simulink model "MideaPMSM_V3_2019A"  (R2019b)
settings: Solver=ode4  StartTime=0.0  StopTime=0.2  FixedStep=1e-6  RelTol=1e-3
InitFcn:
  | Ts = 1e-6;
  | Pn = 3;
undefined symbols (not defined in the file or in its folder): DiscIntNeverNeededParam
libraries: powerlib x24, powerlib_extras x4, simulink x4, powerlib_meascontrol x3, dsparch4 x2
settings Model: Creator=B210b  LastModifiedBy=B210b
settings SFSimCC: CustomCodeUndefinedFunction=UseInterfaceOnly

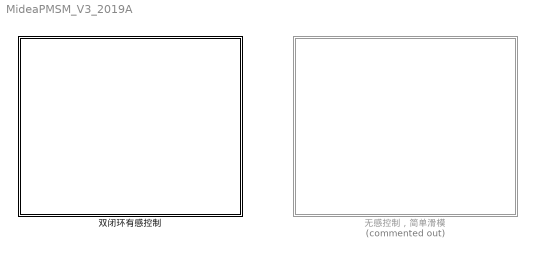
== system MideaPMSM_V3_2019A ==
  双闭环有感控制 : Subsystem
  无感控制，简单滑模 : Subsystem  Commented=on

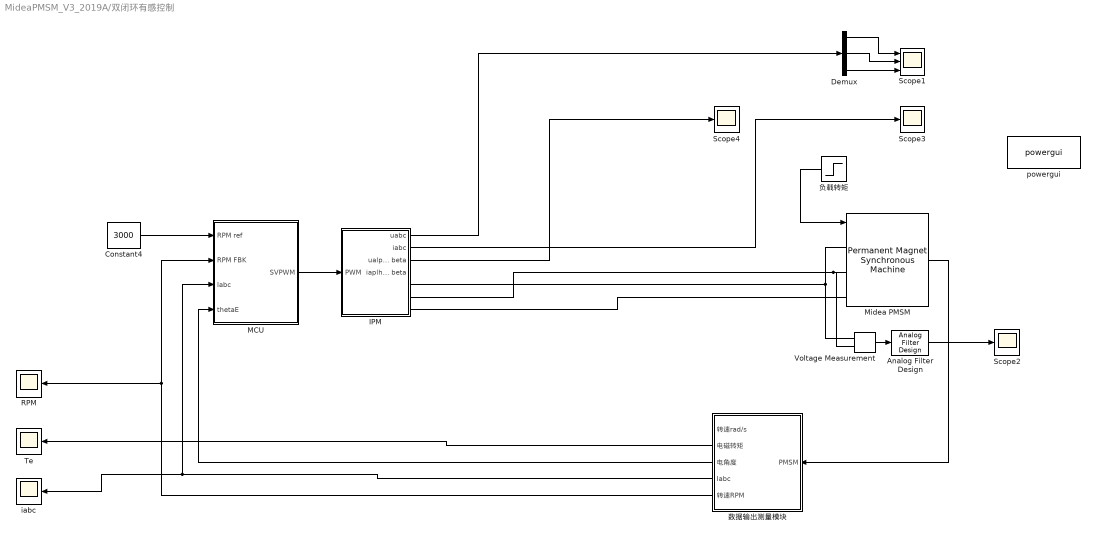
== system MideaPMSM_V3_2019A/双闭环有感控制 ==
  Analog Filter Design : dsparch4/Analog Filter Design  method=Butterworth  filttype=Lowpass  N=2  Wlo=30  Whi=80  Rp=2  Rs=40
  Constant4 : Constant  Value=3000
  Demux : Demux  Outputs=3
  IPM : Subsystem
  MCU : Subsystem
  Midea PMSM : powerlib/Machines/Permanent Magnet Synchronous Machine  NbPhases=3  FluxDistribution=Sinusoidal  RotorType=Salient-pole  MechanicalLoad=Torque Tm  PresetModel=No  ShowDetailedParameters=on  MeasurementBus=off  Resistance=26  Inductance=8.5e-3  dqInductances=[0.066 0.072]  La=0.000835  MachineConstant=Flux linkage established by magnets (V.s)  Flux=0.0714394  VoltageCst=38.873  TorqueCst=0.32148  Flat=120  Mechanical=[3.4e-05 0.000303448 3]  PolePairs=3  InitialConditions=[0,0, 0,0]  InitialConditions5ph=[0 0 0 0 0 0]  RefAngle=Aligned with phase A axis (original Park)  IterativeDiscreteModel=Trapezoidal non iterative  TsBlock=-1  TsPowergui=0
  RPM : Scope
  Scope1 : Scope  NumInputPorts=3
  Scope2 : Scope
  Scope3 : Scope
  Scope4 : Scope
  Te : Scope
  Voltage Measurement : powerlib/Measurements/Voltage Measurement  PhasorSimulation=off  OutputType=Complex  PSBequivalent=0
      settings: SourceProductName=Simscape Electrical
  iabc : Scope
  powergui : powerlib/powergui  SimulationMode=Discrete  SampleTime=1e-6  frequency=60  Iterations=50  frequencyindice=0  Pbase=100e6  ErrMax=1e-4  UnitsV=kV  UnitsW=MW  buscounter=0  FunctionMessages=off  echomessages=off  EnableUseOfTLC=off  CurrentSourceSwitches=on  DisableSnubberDevices=off  DisableRonSwitches=off  DisableVfSwitches=off  DisplayEquations=off  AutomaticDiscreteSolvers=off  SolverType=Tustin/Backward Euler (TBE)  Interpol=off  ExternalGateDelay=off  methode=off  Ts=0  x0status=blocks  SPID=off  SwTol=0  HookPort=off  NonlinearTolerance=1e-4  nMaxIteration=100  ContinueOnMaxIteration=off  RestoreLinks=warning  ResistiveCurrentMeasurement=off  Frange=[0:2:500]  Ylog=off  Xlog=on  ShowGrid=off  save=off  variable=ZData  structure=0  ZoomFFT=on  StartTime=0.0  cycles=1  DisplayStyle=1  fundamental=60  FreqAxis=off  MaxFrequency=1000  frequencyindicesteady=1  RmsSteady=1  display=off
      settings: SourceProductName=Simscape Electrical
  数据输出测量模块 : Subsystem
  负载转矩 : Step  Time=0.1  After=0  SampleTime=0
  wires:
  数据输出测量模块/3(电角度) -> MCU/4(thetaE)
  数据输出测量模块/5(转速RPM) -> MCU/2(RPM FBK), RPM/1
  负载转矩/1 -> Midea PMSM/1
  Midea PMSM/1 -> 数据输出测量模块/1(PMSM)
  数据输出测量模块/2(电磁转矩) -> Te/1
  Constant4/1 -> MCU/1(RPM ref)
  数据输出测量模块/4(Iabc) -> iabc/1, MCU/3(Iabc)
  MCU/1(SVPWM) -> IPM/1(PWM)
  IPM/2(iabc) -> Scope3/1
  IPM/3(ualpha beta) -> Scope4/1
  Demux/1 -> Scope1/1
  Demux/2 -> Scope1/2
  Demux/3 -> Scope1/3
  IPM/1(uabc) -> Demux/1
  Voltage Measurement/1 -> Analog Filter Design/1
  Analog Filter Design/1 -> Scope2/1
  connections:
  IPM/RConn3 -- Midea PMSM/LConn3
  IPM/RConn1 -- Midea PMSM/LConn1 -- Voltage Measurement/LConn1
  IPM/RConn2 -- Voltage Measurement/LConn2 -- Midea PMSM/LConn2

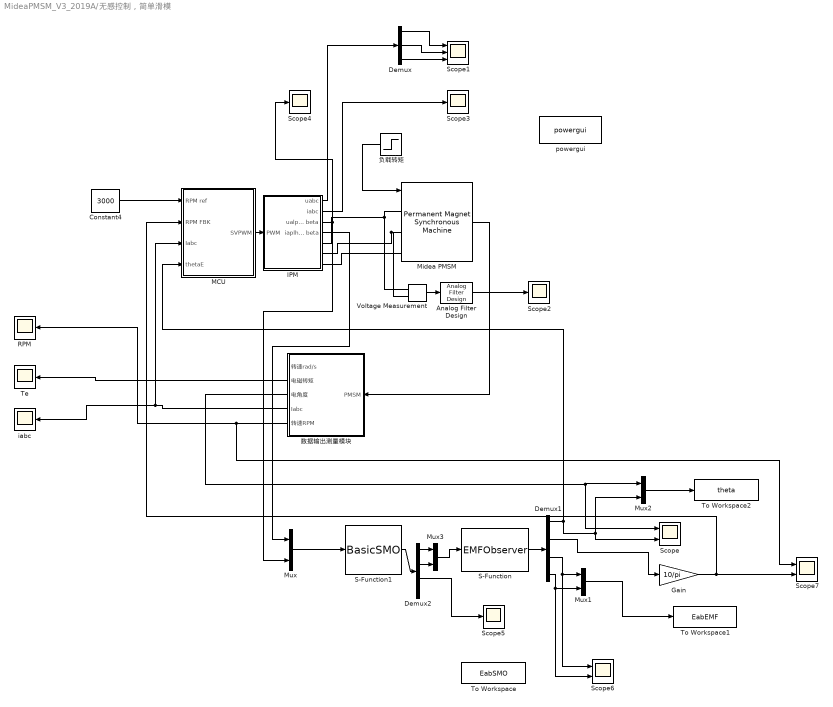
== system MideaPMSM_V3_2019A/无感控制，简单滑模 ==
  Analog Filter Design : dsparch4/Analog Filter Design  method=Butterworth  filttype=Lowpass  N=2  Wlo=30  Whi=80  Rp=2  Rs=40
  Constant4 : Constant  Value=3000
  Demux : Demux  Outputs=3
  Demux1 : Demux
  Demux2 : Demux
  Gain : Gain  Gain=10/pi
  IPM : Subsystem
  MCU : Subsystem
  Midea PMSM : powerlib/Machines/Permanent Magnet Synchronous Machine  NbPhases=3  FluxDistribution=Sinusoidal  RotorType=Round  MechanicalLoad=Torque Tm  PresetModel=No  ShowDetailedParameters=on  MeasurementBus=off  Resistance=26  Inductance=8.5e-3  dqInductances=[0.066 0.072]  La=0.0345  MachineConstant=Flux linkage established by magnets (V.s)  Flux=0.0779697  VoltageCst=42.4264  TorqueCst=0.35086  Flat=120  Mechanical=[3.4e-05 0 3]  PolePairs=3  InitialConditions=[0,0, 0,0]  InitialConditions5ph=[0 0 0 0 0 0]  RefAngle=Aligned with phase A axis (original Park)  IterativeDiscreteModel=Trapezoidal non iterative  TsBlock=-1  TsPowergui=0
  Mux{,1..3} (4 alike) : Mux  Inputs=2
  RPM : Scope
  S-Function : S-Function  FunctionName=EMFObserver  SFunctionDeploymentMode=off  EnableBusSupport=off
  S-Function1 : S-Function  FunctionName=BasicSMO  SFunctionDeploymentMode=off  EnableBusSupport=off
  Scope : Scope  NumInputPorts=2
  Scope1 : Scope  NumInputPorts=3
  Scope{2..5} (4 alike) : Scope
  Scope6 : Scope  NumInputPorts=2
  Scope7 : Scope  NumInputPorts=2
  Te : Scope
  To Workspace : ToWorkspace  VariableName=EabSMO  SaveFormat=Timeseries  SampleTime=-1
  To Workspace1 : ToWorkspace  VariableName=EabEMF  SaveFormat=Timeseries  SampleTime=-1
  To Workspace2 : ToWorkspace  VariableName=theta  SaveFormat=Timeseries  SampleTime=-1
  Voltage Measurement : powerlib/Measurements/Voltage Measurement  PhasorSimulation=off  OutputType=Complex  PSBequivalent=0
      settings: SourceProductName=Simscape Electrical
  iabc : Scope
  powergui : powerlib/powergui  SimulationMode=Discrete  SampleTime=1e-6  frequency=60  Iterations=50  frequencyindice=0  Pbase=100e6  ErrMax=1e-4  UnitsV=kV  UnitsW=MW  buscounter=0  FunctionMessages=off  echomessages=off  EnableUseOfTLC=off  CurrentSourceSwitches=on  DisableSnubberDevices=off  DisableRonSwitches=off  DisableVfSwitches=off  DisplayEquations=off  AutomaticDiscreteSolvers=off  SolverType=Tustin/Backward Euler (TBE)  Interpol=off  ExternalGateDelay=off  methode=off  Ts=0  x0status=blocks  SPID=off  SwTol=0  HookPort=off  NonlinearTolerance=1e-4  nMaxIteration=100  ContinueOnMaxIteration=off  RestoreLinks=warning  ResistiveCurrentMeasurement=off  Frange=[0:2:500]  Ylog=off  Xlog=on  ShowGrid=off  save=off  variable=ZData  structure=0  ZoomFFT=on  StartTime=0.0  cycles=1  DisplayStyle=1  fundamental=60  FreqAxis=off  MaxFrequency=1000  frequencyindicesteady=1  RmsSteady=1  display=off
      settings: SourceProductName=Simscape Electrical
  数据输出测量模块 : Subsystem
  负载转矩 : Step  Time=0.1  After=0.19  SampleTime=0
  wires:
  数据输出测量模块/3(电角度) -> Mux2/1, Scope/1
  负载转矩/1 -> Midea PMSM/1
  Midea PMSM/1 -> 数据输出测量模块/1(PMSM)
  数据输出测量模块/2(电磁转矩) -> Te/1
  Constant4/1 -> MCU/1(RPM ref)
  数据输出测量模块/4(Iabc) -> MCU/3(Iabc), iabc/1
  MCU/1(SVPWM) -> IPM/1(PWM)
  IPM/2(iabc) -> Scope3/1
  IPM/3(ualpha beta) -> Mux/2, Scope4/1
  Demux/1 -> Scope1/1
  Demux/2 -> Scope1/2
  Demux/3 -> Scope1/3
  IPM/1(uabc) -> Demux/1
  Voltage Measurement/1 -> Analog Filter Design/1
  Analog Filter Design/1 -> Scope2/1
  Mux/1 -> S-Function1/1
  IPM/4(iaplha beta) -> Mux/1
  S-Function/1 -> Demux1/1
  Demux1/4 -> Scope6/2, Mux1/2
  Demux1/3 -> Scope6/1, Mux1/1
  Demux1/2 -> Gain/1
  Gain/1 -> MCU/2(RPM FBK), Scope7/2
  Mux1/1 -> To Workspace1/1
  Mux2/1 -> To Workspace2/1
  Demux1/1 -> Scope/2, Mux2/2, MCU/4(thetaE)
  数据输出测量模块/5(转速RPM) -> Scope7/1, RPM/1
  S-Function1/1 -> Demux2/1
  Demux2/1 -> Mux3/1
  Demux2/2 -> Mux3/2
  Mux3/1 -> S-Function/1
  Demux2/3 -> Scope5/1
  connections:
  IPM/RConn3 -- Midea PMSM/LConn3
  IPM/RConn1 -- Midea PMSM/LConn1 -- Voltage Measurement/LConn1
  IPM/RConn2 -- Voltage Measurement/LConn2 -- Midea PMSM/LConn2

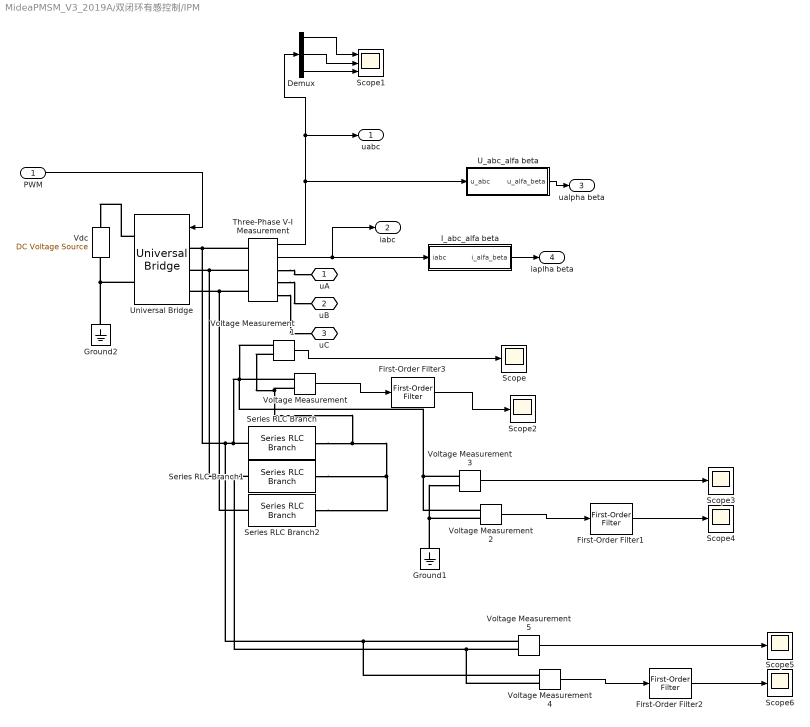
== system MideaPMSM_V3_2019A/双闭环有感控制/IPM ==
  PWM : Inport
  Demux : Demux  Outputs=3
  First-Order Filter1 : powerlib_meascontrol/Filters/First-Order Filter  FilterType=Lowpass  Tc=10e-3  Ts=0  Initialize=on  Vac_Init=[0, 0, 60]  Vdc_Init=0  PlotResponse=off  FreqRange="[0,  200,  1]"
      settings: SourceProductName=Simscape Electrical
  First-Order Filter2 : powerlib_meascontrol/Filters/First-Order Filter  FilterType=Lowpass  Tc=10e-3  Ts=0  Initialize=on  Vac_Init=[0, 0, 60]  Vdc_Init=0  PlotResponse=off  FreqRange="[0,  200,  1]"
      settings: SourceProductName=Simscape Electrical
  First-Order Filter3 : powerlib_meascontrol/Filters/First-Order Filter  FilterType=Lowpass  Tc=10e-3  Ts=0  Initialize=on  Vac_Init=[0, 0, 60]  Vdc_Init=0  PlotResponse=off  FreqRange="[0,  200,  1]"
      settings: SourceProductName=Simscape Electrical
  Ground1 : powerlib/Elements/Ground  LConnTagsString=a
      settings: SourceProductName=Simscape Electrical
  Ground2 : powerlib/Elements/Ground  LConnTagsString=a
      settings: SourceProductName=Simscape Electrical
  I_abc_alfa beta : Subsystem
  Scope{,2..6} (6 alike) : Scope
  Scope1 : Scope  NumInputPorts=3
  Series RLC Branch : powerlib/Elements/Series RLC Branch  LConnTagsString=__new0  RConnTagsString=__new0  BranchType=R  Resistance=5  Inductance=0  SetiL0=off  InitialCurrent=0  Capacitance=0  Setx0=off  InitialVoltage=0  Measurements=None
      settings: SourceProductName=Simscape Electrical
  Series RLC Branch1 : powerlib/Elements/Series RLC Branch  LConnTagsString=__new0  RConnTagsString=__new0  BranchType=R  Resistance=5  Inductance=0  SetiL0=off  InitialCurrent=0  Capacitance=0  Setx0=off  InitialVoltage=0  Measurements=None
      settings: SourceProductName=Simscape Electrical
  Series RLC Branch2 : powerlib/Elements/Series RLC Branch  LConnTagsString=__new0  RConnTagsString=__new0  BranchType=R  Resistance=5  Inductance=0  SetiL0=off  InitialCurrent=0  Capacitance=0  Setx0=off  InitialVoltage=0  Measurements=None
      settings: SourceProductName=Simscape Electrical
  Three-Phase V-I Measurement : powerlib/Measurements/Three-Phase V-I Measurement  VoltageMeasurement=phase-to-ground  SetLabelV=off  LabelV=Vabc  Vpu=off  VpuLL=off  CurrentMeasurement=yes  SetLabelI=off  LabelI=Iabc  Ipu=off  Pbase=100e6  Vbase=500e3  OutputType=Complex  PhasorSimulation=off  PSBequivalent=0
      settings: SourceProductName=Simscape Electrical
  U_abc_alfa beta : Subsystem
  Universal Bridge : powerlib/Power Electronics/Universal Bridge  Arms=3  SnubberResistance=1e5  SnubberCapacitance=inf  Device=IGBT / Diodes  Ron=1e-3  Lon=0  ForwardVoltages="[  0  0  ]"  ForwardVoltage=0  GTOparameters=[ 10e-6 , 20e-6 ]  IGBTparameters=[ 1e-6 , 2e-6 ]  Measurements=None  Measurements_2=None  converterType=Rectifier
      settings: SourceProductName=Simscape Electrical
  Vdc : powerlib/Electrical Sources/DC Voltage Source  Amplitude=311  Measurements=None
      settings: SourceProductName=Simscape Electrical
  Voltage Measurement{,1..5} (6 alike) : powerlib/Measurements/Voltage Measurement  PhasorSimulation=off  OutputType=Complex  PSBequivalent=0
      settings: SourceProductName=Simscape Electrical
  uA : PMIOPort  Side=Right
  uB : PMIOPort  Port=2  Side=Right
  uC : PMIOPort  Port=3  Side=Right
  uabc : Outport
  iabc : Outport  Port=2
  ualpha beta : Outport  Port=3
  iaplha beta : Outport  Port=4
  wires:
  PWM/1 -> Universal Bridge/1
  Three-Phase V-I Measurement/2 -> iabc/1, I_abc_alfa beta/1(iabc)
  I_abc_alfa beta/1(i_alfa_beta) -> iaplha beta/1
  U_abc_alfa beta/1(u_alfa_beta) -> ualpha beta/1
  Three-Phase V-I Measurement/1 -> U_abc_alfa beta/1(u_abc), Demux/1, uabc/1
  Voltage Measurement/1 -> First-Order Filter3/1
  Demux/2 -> Scope1/2
  Demux/1 -> Scope1/1
  Demux/3 -> Scope1/3
  Voltage Measurement1/1 -> Scope/1
  First-Order Filter1/1 -> Scope4/1
  Voltage Measurement3/1 -> Scope3/1
  Voltage Measurement2/1 -> First-Order Filter1/1
  First-Order Filter3/1 -> Scope2/1
  Voltage Measurement4/1 -> First-Order Filter2/1
  Voltage Measurement5/1 -> Scope5/1
  First-Order Filter2/1 -> Scope6/1
  connections:
  Universal Bridge/RConn1 -- Vdc/RConn1
  Universal Bridge/RConn2 -- Ground2/LConn1 -- Vdc/LConn1
  Three-Phase V-I Measurement/LConn1 -- Voltage Measurement4/LConn1 -- Voltage Measurement5/LConn1 -- Voltage Measurement2/LConn1 -- Voltage Measurement3/LConn1 -- Voltage Measurement1/LConn1 -- Voltage Measurement/LConn1 -- Series RLC Branch/LConn1 -- Universal Bridge/LConn1
  Three-Phase V-I Measurement/LConn2 -- Voltage Measurement4/LConn2 -- Voltage Measurement5/LConn2 -- Series RLC Branch1/LConn1 -- Universal Bridge/LConn2
  Three-Phase V-I Measurement/LConn3 -- Series RLC Branch2/LConn1 -- Universal Bridge/LConn3
  Three-Phase V-I Measurement/RConn1 -- uA/RConn1
  Three-Phase V-I Measurement/RConn2 -- uB/RConn1
  Three-Phase V-I Measurement/RConn3 -- uC/RConn1
  Series RLC Branch2/RConn1 -- Voltage Measurement1/LConn2 -- Voltage Measurement/LConn2 -- Series RLC Branch/RConn1 -- Series RLC Branch1/RConn1
  Ground1/LConn1 -- Voltage Measurement2/LConn2 -- Voltage Measurement3/LConn2

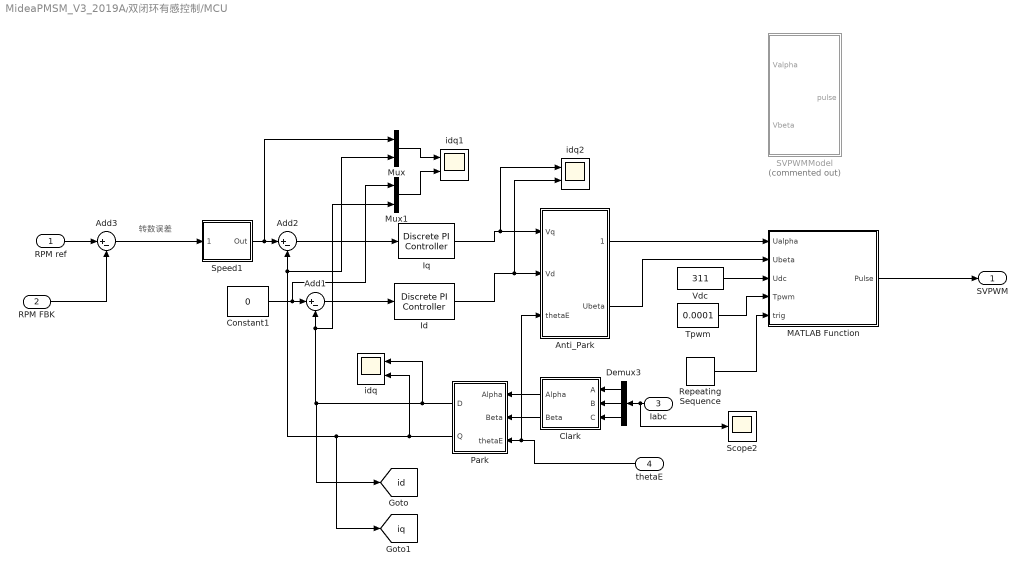
== system MideaPMSM_V3_2019A/双闭环有感控制/MCU ==
  note: 转数误差
  RPM ref : Inport
  RPM FBK : Inport  Port=2
  Iabc : Inport  Port=3
  thetaE : Inport  Port=4
  Add1 : Sum  Inputs=|+-
  Add2 : Sum  Inputs=|+-
  Add3 : Sum  Inputs=|+-
  Anti_Park : Subsystem
  Clark : Subsystem
  Constant1 : Constant  Value=0
  Demux3 : Demux  Outputs=3
  Id : powerlib_extras/Discrete  Control Blocks/Discrete PI Controller  Kp=500  Ki=100000  Par_Limits=[311*0.9*sqrt(3)/2 -311*0.9*sqrt(3)/2]  Init=0  Ts=Ts
      settings: SourceProductName=Simscape Electrical
  Iq : powerlib_extras/Discrete  Control Blocks/Discrete PI Controller  Kp=500  Ki=100000  Par_Limits=[311*0.9*sqrt(3)/2 -311*0.9*sqrt(3)/2]  Init=0  Ts=Ts
      settings: SourceProductName=Simscape Electrical
  MATLAB Function : MATLAB Function  TreatAsAtomicUnit=on
  Mux : Mux  Inputs=2
  Mux1 : Mux  Inputs=2
  Park : Subsystem
  Repeating Sequence : simulink/Sources/Repeating Sequence  rep_seq_t=[0 0.00005 0.0001]  rep_seq_y=[0 0.00005 0]
  SVPWMModel : Subsystem  Commented=on
  Scope2 : Scope
  Speed1 : Subsystem  AncestorBlock=|  DialogController=POWERSYS.PowerSysDialog  mask(Discrete PI Controller){Kpw=0.01, Kiw=2, Ba=0, Par_Limits=[2 -2], Init=0, Ts=-1}
      | powerlib_extras/Discrete 
      | Control Blocks/Discrete
      | PI Controller
      mask prompts: Kpw "Proportional gain (Kp):"; Kiw "Integral gain (Ki):"; Ba "feedback gain (Ba)"; Par_Limits "Output limits: [ Upper   Lower ]"; Init "Output initial value:"; Ts "Sample time:"
      mask help: This block implements a discrete PI controller.
      mask init:
      | UpperLimit=Par_Limits(1);
      | LowerLimit=Par_Limits(2);
      | power_initmask();
      mask Help: This block is part of a subset of blocks in the Extras library that does not have documentation associated with it, other than the block mask description.
      mask Display: disp('PI');
  Tpwm : Constant  Value=0.0001
  Vdc : Constant  Value=311
  idq : Scope  NumInputPorts=2
  idq1 : Scope  NumInputPorts=2
  idq2 : Scope  NumInputPorts=2
  SVPWM : Outport
  tag scope: id=global, iq=global
  wires:
  Clark/1(Alpha) -> Park/1(Alpha)
  Add1/1 -> Id/1
  Park/1(D) -> idq/1, [id], Mux1/2, Add1/2
  Iq/1 -> idq2/1, Anti_Park/1(Vq)
  Speed1/1(Out) -> Mux/1, Add2/1
  Park/2(Q) -> idq/2, [iq], Mux/2, Add2/2
  Id/1 -> idq2/2, Anti_Park/2(Vd)
  Demux3/3 -> Clark/3(C)
  Clark/2(Beta) -> Park/2(Beta)
  thetaE/1 -> Anti_Park/3(thetaE), Park/3(thetaE)
  Add2/1 -> Iq/1
  Demux3/1 -> Clark/1(A)
  Constant1/1 -> Mux1/1, Add1/1
  Demux3/2 -> Clark/2(B)
  Add3/1 -> Speed1/1(Error)
  Iabc/1 -> Scope2/1, Demux3/1
  RPM ref/1 -> Add3/1
  RPM FBK/1 -> Add3/2
  Mux/1 -> idq1/1
  Mux1/1 -> idq1/2
  Vdc/1 -> MATLAB Function/3(Udc)
  Tpwm/1 -> MATLAB Function/4(Tpwm)
  Anti_Park/1(Ualpha) -> MATLAB Function/1(Ualpha)
  Anti_Park/2(Ubeta) -> MATLAB Function/2(Ubeta)
  MATLAB Function/1(Pulse) -> SVPWM/1
  Repeating Sequence/1 -> MATLAB Function/5(trig)

== system MideaPMSM_V3_2019A/双闭环有感控制/数据输出测量模块 ==
  PMSM : Inport
  Mux : Subsystem
  Pn : Gain  Gain=Pn
  Scope : Scope  NumInputPorts=2
  wm->Nr : Gain  Gain=30/pi
  转速rad/s : Outport
  电磁转矩 : Outport  Port=2
  电角度 : Outport  Port=3
  Iabc : Outport  Port=4
  转速RPM : Outport  Port=5
  wires:
  Mux/1(Te) -> 电磁转矩/1
  Mux/2(The) -> Pn/1
  PMSM/1 -> Mux/1(m)
  Mux/4(Wm) -> wm->Nr/1, 转速rad/s/1
  Pn/1 -> 电角度/1
  Mux/3(Iabc) -> Iabc/1
  wm->Nr/1 -> 转速RPM/1
  Mux/5(vd) -> Scope/1
  Mux/6(vq) -> Scope/2

== system MideaPMSM_V3_2019A/无感控制，简单滑模/IPM ==
  PWM : Inport
  Ground2 : powerlib/Elements/Ground  LConnTagsString=a
      settings: SourceProductName=Simscape Electrical
  I_abc_alfa beta : Subsystem
  Three-Phase V-I Measurement : powerlib/Measurements/Three-Phase V-I Measurement  VoltageMeasurement=phase-to-ground  SetLabelV=off  LabelV=Vabc  Vpu=off  VpuLL=off  CurrentMeasurement=yes  SetLabelI=off  LabelI=Iabc  Ipu=off  Pbase=100e6  Vbase=500e3  OutputType=Complex  PhasorSimulation=off  PSBequivalent=0
      settings: SourceProductName=Simscape Electrical
  U_abc_alfa beta : Subsystem
  Universal Bridge : powerlib/Power Electronics/Universal Bridge  Arms=3  SnubberResistance=1e5  SnubberCapacitance=inf  Device=IGBT / Diodes  Ron=1e-3  Lon=0  ForwardVoltages="[  0  0  ]"  ForwardVoltage=0  GTOparameters=[ 10e-6 , 20e-6 ]  IGBTparameters=[ 1e-6 , 2e-6 ]  Measurements=None  Measurements_2=None  converterType=Rectifier
      settings: SourceProductName=Simscape Electrical
  Vdc : powerlib/Electrical Sources/DC Voltage Source  Amplitude=311  Measurements=None
      settings: SourceProductName=Simscape Electrical
  uA : PMIOPort  Side=Right
  uB : PMIOPort  Port=2  Side=Right
  uC : PMIOPort  Port=3  Side=Right
  uabc : Outport
  iabc : Outport  Port=2
  ualpha beta : Outport  Port=3
  iaplha beta : Outport  Port=4
  wires:
  PWM/1 -> Universal Bridge/1
  Three-Phase V-I Measurement/2 -> iabc/1, I_abc_alfa beta/1(iabc)
  I_abc_alfa beta/1(i_alfa_beta) -> iaplha beta/1
  U_abc_alfa beta/1(u_alfa_beta) -> ualpha beta/1
  Three-Phase V-I Measurement/1 -> U_abc_alfa beta/1(u_abc), uabc/1
  connections:
  Universal Bridge/RConn1 -- Vdc/RConn1
  Universal Bridge/RConn2 -- Ground2/LConn1 -- Vdc/LConn1
  Three-Phase V-I Measurement/LConn1 -- Universal Bridge/LConn1
  Three-Phase V-I Measurement/LConn2 -- Universal Bridge/LConn2
  Three-Phase V-I Measurement/LConn3 -- Universal Bridge/LConn3
  Three-Phase V-I Measurement/RConn1 -- uA/RConn1
  Three-Phase V-I Measurement/RConn2 -- uB/RConn1
  Three-Phase V-I Measurement/RConn3 -- uC/RConn1

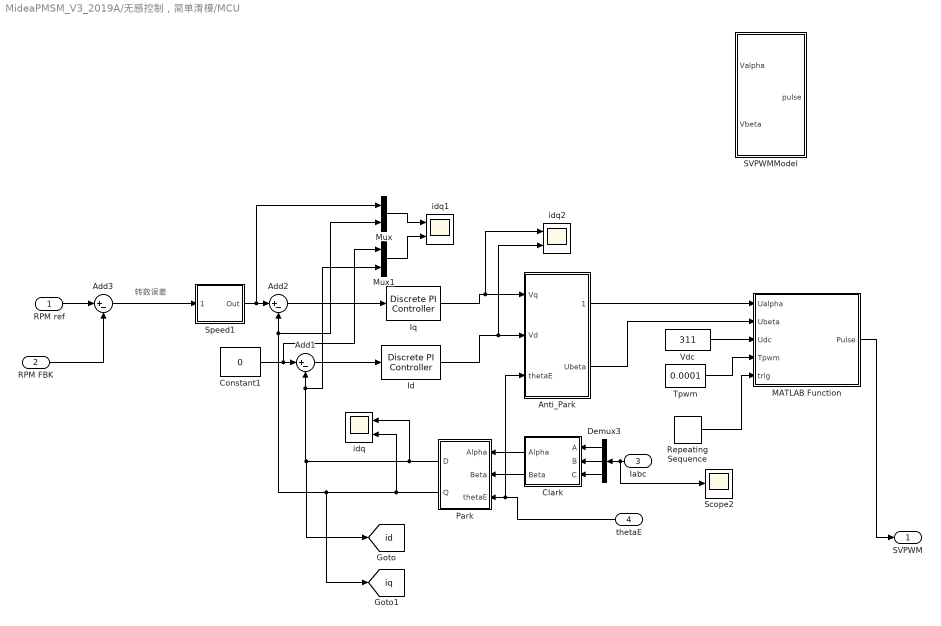
== system MideaPMSM_V3_2019A/无感控制，简单滑模/MCU ==
  note: 转数误差
  RPM ref : Inport
  RPM FBK : Inport  Port=2
  Iabc : Inport  Port=3
  thetaE : Inport  Port=4
  Add1 : Sum  Inputs=|+-
  Add2 : Sum  Inputs=|+-
  Add3 : Sum  Inputs=|+-
  Anti_Park : Subsystem
  Clark : Subsystem
  Constant1 : Constant  Value=0
  Demux3 : Demux  Outputs=3
  Id : powerlib_extras/Discrete  Control Blocks/Discrete PI Controller  Kp=500  Ki=100000  Par_Limits=[311*0.9*sqrt(3)/2 -311*0.9*sqrt(3)/2]  Init=0  Ts=Ts
      settings: SourceProductName=Simscape Electrical
  Iq : powerlib_extras/Discrete  Control Blocks/Discrete PI Controller  Kp=500  Ki=100000  Par_Limits=[311*0.9*sqrt(3)/2 -311*0.9*sqrt(3)/2]  Init=0  Ts=Ts
      settings: SourceProductName=Simscape Electrical
  MATLAB Function : MATLAB Function  TreatAsAtomicUnit=on
  Mux : Mux  Inputs=2
  Mux1 : Mux  Inputs=2
  Park : Subsystem
  Repeating Sequence : simulink/Sources/Repeating Sequence  rep_seq_t=[0 0.00005 0.0001]  rep_seq_y=[0 0.00005 0]
  SVPWMModel : Subsystem
  Scope2 : Scope
  Speed1 : Subsystem  AncestorBlock=|  DialogController=POWERSYS.PowerSysDialog  mask(Discrete PI Controller){Kpw=0.01, Kiw=2, Ba=0, Par_Limits=[2 -2], Init=0, Ts=-1}
      | powerlib_extras/Discrete 
      | Control Blocks/Discrete
      | PI Controller
      mask prompts: Kpw "Proportional gain (Kp):"; Kiw "Integral gain (Ki):"; Ba "feedback gain (Ba)"; Par_Limits "Output limits: [ Upper   Lower ]"; Init "Output initial value:"; Ts "Sample time:"
      mask help: This block implements a discrete PI controller.
      mask init:
      | UpperLimit=Par_Limits(1);
      | LowerLimit=Par_Limits(2);
      | power_initmask();
      mask Help: This block is part of a subset of blocks in the Extras library that does not have documentation associated with it, other than the block mask description.
      mask Display: disp('PI');
  Tpwm : Constant  Value=0.0001
  Vdc : Constant  Value=311
  idq : Scope  NumInputPorts=2
  idq1 : Scope  NumInputPorts=2
  idq2 : Scope  NumInputPorts=2
  SVPWM : Outport
  tag scope: id=global, iq=global
  wires:
  Clark/1(Alpha) -> Park/1(Alpha)
  Add1/1 -> Id/1
  Park/1(D) -> idq/1, [id], Mux1/2, Add1/2
  Iq/1 -> idq2/1, Anti_Park/1(Vq)
  Speed1/1(Out) -> Mux/1, Add2/1
  Park/2(Q) -> idq/2, [iq], Mux/2, Add2/2
  Id/1 -> idq2/2, Anti_Park/2(Vd)
  Demux3/3 -> Clark/3(C)
  Clark/2(Beta) -> Park/2(Beta)
  thetaE/1 -> Anti_Park/3(thetaE), Park/3(thetaE)
  Add2/1 -> Iq/1
  Demux3/1 -> Clark/1(A)
  Constant1/1 -> Mux1/1, Add1/1
  Demux3/2 -> Clark/2(B)
  Add3/1 -> Speed1/1(Error)
  Iabc/1 -> Scope2/1, Demux3/1
  RPM ref/1 -> Add3/1
  RPM FBK/1 -> Add3/2
  Mux/1 -> idq1/1
  Mux1/1 -> idq1/2
  Repeating Sequence/1 -> MATLAB Function/5(trig)
  Vdc/1 -> MATLAB Function/3(Udc)
  Tpwm/1 -> MATLAB Function/4(Tpwm)
  Anti_Park/1(Ualpha) -> MATLAB Function/1(Ualpha)
  Anti_Park/2(Ubeta) -> MATLAB Function/2(Ubeta)
  MATLAB Function/1(Pulse) -> SVPWM/1

== system MideaPMSM_V3_2019A/无感控制，简单滑模/数据输出测量模块 ==
  PMSM : Inport
  Constant : Constant  Value=2*pi
  Math Function : Math  Operator=rem  SignedPower=off  SaturateOnIntegerOverflow=on
  Mux : Subsystem
  Pn : Gain  Gain=Pn
  Scope : Scope  NumInputPorts=2
  wm->Nr : Gain  Gain=30/pi
  转速rad/s : Outport
  电磁转矩 : Outport  Port=2
  电角度 : Outport  Port=3
  Iabc : Outport  Port=4
  转速RPM : Outport  Port=5
  wires:
  Mux/1(Te) -> 电磁转矩/1
  Mux/2(The) -> Pn/1
  PMSM/1 -> Mux/1(m)
  Mux/4(Wm) -> wm->Nr/1, 转速rad/s/1
  Mux/3(Iabc) -> Iabc/1
  wm->Nr/1 -> 转速RPM/1
  Mux/5(vd) -> Scope/1
  Mux/6(vq) -> Scope/2
  Math Function/1 -> 电角度/1
  Pn/1 -> Math Function/1
  Constant/1 -> Math Function/2

== system MideaPMSM_V3_2019A/双闭环有感控制/IPM/I_abc_alfa beta ==
  iabc : Inport
  Fcn : Fcn  Expr=(2*u(1)-u(2)-u(3))/3
  Fcn1 : Fcn  Expr=(u(2)-u(3))/(3^(1/2))
  Mux2 : Mux  Inputs=2
  i_alfa_beta : Outport
  wires:
  iabc/1 -> Fcn/1, Fcn1/1
  Mux2/1 -> i_alfa_beta/1
  Fcn/1 -> Mux2/1
  Fcn1/1 -> Mux2/2

== system MideaPMSM_V3_2019A/双闭环有感控制/IPM/U_abc_alfa beta ==
  u_abc : Inport
  Fcn : Fcn  Expr=(2*u(1)-u(2)-u(3))/3
  Fcn1 : Fcn  Expr=(u(2)-u(3))/(3^(1/2))
  Mux2 : Mux  Inputs=2
  u_alfa_beta : Outport
  wires:
  u_abc/1 -> Fcn/1, Fcn1/1
  Mux2/1 -> u_alfa_beta/1
  Fcn/1 -> Mux2/1
  Fcn1/1 -> Mux2/2

== system MideaPMSM_V3_2019A/双闭环有感控制/MCU/Anti_Park ==
  Vq : Inport
  Vd : Inport  Port=2
  thetaE : Inport  Port=3
  Fcn : Fcn  Expr=cos(u[1])*u[2]-sin(u[1])*u[3]
  Fcn1 : Fcn  Expr=sin(u[1])*u[2]+cos(u[1])*u[3]
  Mux1 : Mux  Inputs=3
  Ualpha : Outport
  Ubeta : Outport  Port=2
  wires:
  Fcn1/1 -> Ubeta/1
  Fcn/1 -> Ualpha/1
  Mux1/1 -> Fcn/1, Fcn1/1
  Vd/1 -> Mux1/2
  Vq/1 -> Mux1/3
  thetaE/1 -> Mux1/1

== system MideaPMSM_V3_2019A/双闭环有感控制/MCU/Clark ==
  A : Inport
  B : Inport  Port=2
  C : Inport  Port=3
  Mux : Mux  Inputs=3
  alpha : Fcn  Expr=(u(1)-0.5*(u(2)+u(3)))*2/3
  beta : Fcn  Expr=sqrt(3)/2*(u(2)-u(3))*2/3
  Alpha : Outport
  Beta : Outport  Port=2
  wires:
  alpha/1 -> Alpha/1
  B/1 -> Mux/2
  C/1 -> Mux/3
  A/1 -> Mux/1
  Mux/1 -> beta/1, alpha/1
  beta/1 -> Beta/1

== system MideaPMSM_V3_2019A/双闭环有感控制/MCU/Park ==
  Alpha : Inport
  Beta : Inport  Port=2
  thetaE : Inport  Port=3
  Mux : Mux  Inputs=3
  d : Fcn  Expr=u(1)*cos(u(3))+u(2)*sin(u(3))
  q : Fcn  Expr=-u(1)*sin(u(3))+u(2)*cos(u(3))
  D : Outport
  Q : Outport  Port=2
  wires:
  d/1 -> D/1
  Beta/1 -> Mux/2
  Alpha/1 -> Mux/1
  Mux/1 -> q/1, d/1
  q/1 -> Q/1
  thetaE/1 -> Mux/3

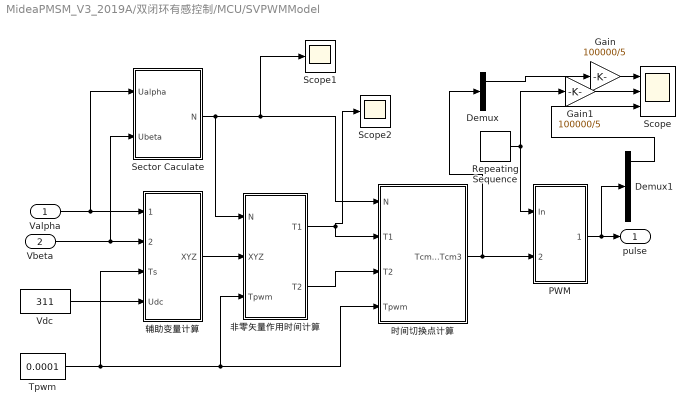
== system MideaPMSM_V3_2019A/双闭环有感控制/MCU/SVPWMModel ==
  Valpha : Inport
  Vbeta : Inport  Port=2
  Demux : Demux  Outputs=3
  Demux1 : Demux  Outputs=6
  Gain : Gain  Gain=100000/5
  Gain1 : Gain  Gain=100000/5
  PWM : Subsystem
  Repeating Sequence : simulink/Sources/Repeating Sequence  rep_seq_t=[0 0.00005 0.0001]  rep_seq_y=[0 0.00005 0]
  Scope : Scope  NumInputPorts=3
  Scope1 : Scope
  Scope2 : Scope
  Sector Caculate : Subsystem
  Tpwm : Constant  Value=0.0001
  Vdc : Constant  Value=311
  时间切换点计算 : Subsystem
  辅助变量计算 : Subsystem
  非零矢量作用时间计算 : Subsystem
  pulse : Outport
  wires:
  PWM/1(PWM) -> Demux1/1, pulse/1
  Repeating Sequence/1 -> Gain1/1, PWM/1(In)
  Vbeta/1 -> 辅助变量计算/2(Ubeta), Sector Caculate/2(Ubeta)
  非零矢量作用时间计算/1(T1) -> 时间切换点计算/2(T1), Scope2/1
  Valpha/1 -> 辅助变量计算/1(Ualpha), Sector Caculate/1(Ualpha)
  非零矢量作用时间计算/2(T2) -> 时间切换点计算/3(T2)
  Sector Caculate/1("N ") -> Scope1/1, 时间切换点计算/1(N), 非零矢量作用时间计算/1(N)
  辅助变量计算/1(XYZ) -> 非零矢量作用时间计算/2(XYZ)
  Tpwm/1 -> 辅助变量计算/3(Ts), 时间切换点计算/4(Tpwm), 非零矢量作用时间计算/3(Tpwm)
  Vdc/1 -> 辅助变量计算/4(Udc)
  时间切换点计算/1(Tcm1 Tcm2 Tcm3) -> PWM/2(Tcm123), Demux/1
  Demux/1 -> Gain/1
  Demux1/1 -> Scope/3
  Gain1/1 -> Scope/2
  Gain/1 -> Scope/1

== system MideaPMSM_V3_2019A/双闭环有感控制/MCU/Speed1 ==
  note: Discrete PID Controller
  note: Pierre Giroux, Gilbert Sybille
      | Power System Simulation Laboratory
      | IREQ, Hydro-Quebc
  Error : Inport  SampleTime=Ts
  Discrete-Time Integrator : DiscreteIntegrator  InitialCondition=Init  SampleTime=Ts  LimitOutput=on  UpperSaturationLimit=UpperLimit  LowerSaturationLimit=LowerLimit  ICPrevOutput=DiscIntNeverNeededParam  ICPrevScaledInput=DiscIntNeverNeededParam
  Kp1 : Gain  Gain=Ba  SampleTime=Ts  SaturateOnIntegerOverflow=on  OutDataTypeStr=Inherit: Same as input  ParamDataTypeStr=Inherit: Same as input
  Kp4 : Gain  Gain=Kpw  SampleTime=Ts  SaturateOnIntegerOverflow=on  OutDataTypeStr=Inherit: Same as input  ParamDataTypeStr=Inherit: Same as input
  Kp5 : Gain  Gain=Kiw  SampleTime=Ts  SaturateOnIntegerOverflow=on  OutDataTypeStr=Inherit: Same as input  ParamDataTypeStr=Inherit: Same as input
  Saturation2 : Saturate  UpperLimit=UpperLimit  LowerLimit=LowerLimit  SampleTime=Ts
  Sum6 : Sum  Inputs=++-  SampleTime=Ts  SaturateOnIntegerOverflow=on  InputSameDT=on  OutDataTypeStr=Inherit: Same as first input
  Zero-Order Hold : ZeroOrderHold  SampleTime=Ts
  Out : Outport  SampleTime=Ts  InitialOutput=0
  wires:
  Error/1 -> Kp1/1, Kp5/1, Kp4/1
  Zero-Order Hold/1 -> Sum6/1
  Saturation2/1 -> Out/1
  Discrete-Time Integrator/1 -> Sum6/2
  Kp4/1 -> Zero-Order Hold/1
  Kp5/1 -> Discrete-Time Integrator/1
  Sum6/1 -> Saturation2/1
  Kp1/1 -> Sum6/3

== system MideaPMSM_V3_2019A/双闭环有感控制/数据输出测量模块/Mux ==
  m : Inport
  Bus Selector : BusSelector  OutputSignals=Stator current is_a (A),Stator current is_b (A),Stator current is_c (A),Stator voltage Vs_q (V),Stator voltage Vs_d (V)
  Bus Selector1 : BusSelector  OutputSignals=Rotor speed wm (rad/s),Rotor angle thetam (rad),Electromagnetic torque Te (N*m)
  Mux : Mux  Inputs=3
  Te : Outport
  The : Outport  Port=2
  Iabc : Outport  Port=3
  Wm : Outport  Port=4
  vd : Outport  Port=5
  vq : Outport  Port=6
  wires:
  Bus Selector1/1 -> Wm/1  "<Rotor speed wm (rad/s)>"
  Bus Selector1/2 -> The/1  "<Rotor angle thetam (rad)>"
  Bus Selector1/3 -> Te/1  "<Electromagnetic torque Te (N*m)>"
  m/1 -> Bus Selector/1, Bus Selector1/1
  Bus Selector/2 -> Mux/2  "<Stator current is_b (A)>"
  Bus Selector/3 -> Mux/3  "<Stator current is_c (A)>"
  Bus Selector/1 -> Mux/1  "<Stator current is_a (A)>"
  Mux/1 -> Iabc/1
  Bus Selector/4 -> vq/1  "<Stator voltage Vs_q (V)>"
  Bus Selector/5 -> vd/1  "<Stator voltage Vs_d (V)>"

== system MideaPMSM_V3_2019A/无感控制，简单滑模/IPM/I_abc_alfa beta ==
  iabc : Inport
  Fcn : Fcn  Expr=(2*u(1)-u(2)-u(3))/3
  Fcn1 : Fcn  Expr=(u(2)-u(3))/(3^(1/2))
  Mux2 : Mux  Inputs=2
  i_alfa_beta : Outport
  wires:
  iabc/1 -> Fcn/1, Fcn1/1
  Mux2/1 -> i_alfa_beta/1
  Fcn/1 -> Mux2/1
  Fcn1/1 -> Mux2/2

== system MideaPMSM_V3_2019A/无感控制，简单滑模/IPM/U_abc_alfa beta ==
  u_abc : Inport
  Fcn : Fcn  Expr=(2*u(1)-u(2)-u(3))/3
  Fcn1 : Fcn  Expr=(u(2)-u(3))/(3^(1/2))
  Mux2 : Mux  Inputs=2
  u_alfa_beta : Outport
  wires:
  u_abc/1 -> Fcn/1, Fcn1/1
  Mux2/1 -> u_alfa_beta/1
  Fcn/1 -> Mux2/1
  Fcn1/1 -> Mux2/2

== system MideaPMSM_V3_2019A/无感控制，简单滑模/MCU/Anti_Park ==
  Vq : Inport
  Vd : Inport  Port=2
  thetaE : Inport  Port=3
  Fcn : Fcn  Expr=cos(u[1])*u[2]-sin(u[1])*u[3]
  Fcn1 : Fcn  Expr=sin(u[1])*u[2]+cos(u[1])*u[3]
  Mux1 : Mux  Inputs=3
  Ualpha : Outport
  Ubeta : Outport  Port=2
  wires:
  Fcn1/1 -> Ubeta/1
  Fcn/1 -> Ualpha/1
  Mux1/1 -> Fcn/1, Fcn1/1
  Vd/1 -> Mux1/2
  Vq/1 -> Mux1/3
  thetaE/1 -> Mux1/1

== system MideaPMSM_V3_2019A/无感控制，简单滑模/MCU/Clark ==
  A : Inport
  B : Inport  Port=2
  C : Inport  Port=3
  Mux : Mux  Inputs=3
  alpha : Fcn  Expr=(u(1)-0.5*(u(2)+u(3)))*2/3
  beta : Fcn  Expr=sqrt(3)/2*(u(2)-u(3))*2/3
  Alpha : Outport
  Beta : Outport  Port=2
  wires:
  alpha/1 -> Alpha/1
  B/1 -> Mux/2
  C/1 -> Mux/3
  A/1 -> Mux/1
  Mux/1 -> beta/1, alpha/1
  beta/1 -> Beta/1

== system MideaPMSM_V3_2019A/无感控制，简单滑模/MCU/Park ==
  Alpha : Inport
  Beta : Inport  Port=2
  thetaE : Inport  Port=3
  Mux : Mux  Inputs=3
  d : Fcn  Expr=u(1)*cos(u(3))+u(2)*sin(u(3))
  q : Fcn  Expr=-u(1)*sin(u(3))+u(2)*cos(u(3))
  D : Outport
  Q : Outport  Port=2
  wires:
  d/1 -> D/1
  Beta/1 -> Mux/2
  Alpha/1 -> Mux/1
  Mux/1 -> q/1, d/1
  q/1 -> Q/1
  thetaE/1 -> Mux/3

== system MideaPMSM_V3_2019A/无感控制，简单滑模/MCU/SVPWMModel ==
  Valpha : Inport
  Vbeta : Inport  Port=2
  PWM : Subsystem
  Repeating Sequence : simulink/Sources/Repeating Sequence  rep_seq_t=[0 0.00005 0.0001]  rep_seq_y=[0 0.00005 0]
  Sector Calculate : Subsystem
  T1T2 Calculate : Subsystem
  Tcm Calculate : Subsystem
  Tpwm : Constant  Value=0.0001
  Vdc : Constant  Value=311
  XYZ Calculate : Subsystem
  pulse : Outport
  wires:
  PWM/1(PWM) -> pulse/1
  Repeating Sequence/1 -> PWM/1(In)
  Vbeta/1 -> XYZ Calculate/2(Ubeta), Sector Calculate/2(Ubeta)
  T1T2 Calculate/1(T1) -> Tcm Calculate/2(T1)
  Valpha/1 -> XYZ Calculate/1(Ualpha), Sector Calculate/1(Ualpha)
  T1T2 Calculate/2(T2) -> Tcm Calculate/3(T2)
  Sector Calculate/1("N ") -> Tcm Calculate/1(N), T1T2 Calculate/1(N)
  XYZ Calculate/1(XYZ) -> T1T2 Calculate/2(XYZ)
  Tpwm/1 -> XYZ Calculate/3(Ts), Tcm Calculate/4(Tpwm), T1T2 Calculate/3(Tpwm)
  Vdc/1 -> XYZ Calculate/4(Udc)
  Tcm Calculate/1(Tcm1 Tcm2 Tcm3) -> PWM/2(Tcm123)

== system MideaPMSM_V3_2019A/无感控制，简单滑模/MCU/Speed1 ==
  note: Discrete PID Controller
  note: Pierre Giroux, Gilbert Sybille
      | Power System Simulation Laboratory
      | IREQ, Hydro-Quebc
  Error : Inport  SampleTime=Ts
  Discrete-Time Integrator : DiscreteIntegrator  InitialCondition=Init  SampleTime=Ts  LimitOutput=on  UpperSaturationLimit=UpperLimit  LowerSaturationLimit=LowerLimit  ICPrevOutput=DiscIntNeverNeededParam  ICPrevScaledInput=DiscIntNeverNeededParam
  Kp1 : Gain  Gain=Ba  SampleTime=Ts  SaturateOnIntegerOverflow=on  OutDataTypeStr=Inherit: Same as input  ParamDataTypeStr=Inherit: Same as input
  Kp4 : Gain  Gain=Kpw  SampleTime=Ts  SaturateOnIntegerOverflow=on  OutDataTypeStr=Inherit: Same as input  ParamDataTypeStr=Inherit: Same as input
  Kp5 : Gain  Gain=Kiw  SampleTime=Ts  SaturateOnIntegerOverflow=on  OutDataTypeStr=Inherit: Same as input  ParamDataTypeStr=Inherit: Same as input
  Saturation2 : Saturate  UpperLimit=UpperLimit  LowerLimit=LowerLimit  SampleTime=Ts
  Sum6 : Sum  Inputs=++-  SampleTime=Ts  SaturateOnIntegerOverflow=on  InputSameDT=on  OutDataTypeStr=Inherit: Same as first input
  Zero-Order Hold : ZeroOrderHold  SampleTime=Ts
  Out : Outport  SampleTime=Ts  InitialOutput=0
  wires:
  Error/1 -> Kp1/1, Kp5/1, Kp4/1
  Zero-Order Hold/1 -> Sum6/1
  Saturation2/1 -> Out/1
  Discrete-Time Integrator/1 -> Sum6/2
  Kp4/1 -> Zero-Order Hold/1
  Kp5/1 -> Discrete-Time Integrator/1
  Sum6/1 -> Saturation2/1
  Kp1/1 -> Sum6/3

== system MideaPMSM_V3_2019A/无感控制，简单滑模/数据输出测量模块/Mux ==
  m : Inport
  Bus Selector : BusSelector  OutputSignals=Stator current is_a (A),Stator current is_b (A),Stator current is_c (A),Stator voltage Vs_q (V),Stator voltage Vs_d (V)
  Bus Selector1 : BusSelector  OutputSignals=Rotor speed wm (rad/s),Rotor angle thetam (rad),Electromagnetic torque Te (N*m)
  Mux : Mux  Inputs=3
  Te : Outport
  The : Outport  Port=2
  Iabc : Outport  Port=3
  Wm : Outport  Port=4
  vd : Outport  Port=5
  vq : Outport  Port=6
  wires:
  Bus Selector1/1 -> Wm/1  "<Rotor speed wm (rad/s)>"
  Bus Selector1/2 -> The/1  "<Rotor angle thetam (rad)>"
  Bus Selector1/3 -> Te/1  "<Electromagnetic torque Te (N*m)>"
  m/1 -> Bus Selector/1, Bus Selector1/1
  Bus Selector/2 -> Mux/2  "<Stator current is_b (A)>"
  Bus Selector/3 -> Mux/3  "<Stator current is_c (A)>"
  Bus Selector/1 -> Mux/1  "<Stator current is_a (A)>"
  Mux/1 -> Iabc/1
  Bus Selector/4 -> vq/1  "<Stator voltage Vs_q (V)>"
  Bus Selector/5 -> vd/1  "<Stator voltage Vs_d (V)>"

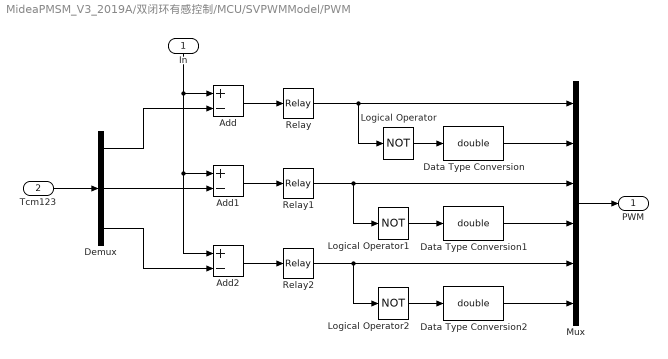
== system MideaPMSM_V3_2019A/双闭环有感控制/MCU/SVPWMModel/PWM ==
  In : Inport
  Tcm123 : Inport  Port=2
  Add : Sum  Inputs=+-
  Add1 : Sum  Inputs=+-
  Add2 : Sum  Inputs=+-
  Data Type Conversion : DataTypeConversion  OutDataTypeStr=double
  Data Type Conversion1 : DataTypeConversion  OutDataTypeStr=double
  Data Type Conversion2 : DataTypeConversion  OutDataTypeStr=double
  Demux : Demux  Outputs=3
  Logical Operator : Logic  Operator=NOT  AllPortsSameDT=off  OutDataTypeStr=boolean
  Logical Operator1 : Logic  Operator=NOT  AllPortsSameDT=off  OutDataTypeStr=boolean
  Logical Operator2 : Logic  Operator=NOT  AllPortsSameDT=off  OutDataTypeStr=boolean
  Mux : Mux  Inputs=6
  Relay : Relay  OffSwitchValue=-eps
  Relay1 : Relay  OffSwitchValue=-eps
  Relay2 : Relay  OffSwitchValue=-eps
  PWM : Outport
  wires:
  Demux/3 -> Add2/2
  Demux/2 -> Add1/2
  Demux/1 -> Add/2
  Relay2/1 -> Mux/5, Logical Operator2/1
  Relay1/1 -> Mux/3, Logical Operator1/1
  Relay/1 -> Logical Operator/1, Mux/1
  Mux/1 -> PWM/1
  Data Type Conversion/1 -> Mux/2
  Data Type Conversion1/1 -> Mux/4
  Data Type Conversion2/1 -> Mux/6
  Logical Operator2/1 -> Data Type Conversion2/1
  Logical Operator1/1 -> Data Type Conversion1/1
  Logical Operator/1 -> Data Type Conversion/1
  Add1/1 -> Relay1/1
  Add2/1 -> Relay2/1
  Add/1 -> Relay/1
  In/1 -> Add/1, Add2/1, Add1/1
  Tcm123/1 -> Demux/1

== system MideaPMSM_V3_2019A/双闭环有感控制/MCU/SVPWMModel/Sector Caculate ==
  Ualpha : Inport
  Ubeta : Inport  Port=2
  B0 : Fcn  Expr=u[2]
  B1 : Fcn  Expr=u[1]*sqrt(3/4)-0.5*u[2]
  B2 : Fcn  Expr=-u[1]*sqrt(3/4)-u[2]*0.5
  Constant : Constant
  Constant1 : Constant  Value=0
  Mux : Mux  Inputs=2
  Mux1 : Mux  Inputs=3
  N : Fcn  Expr=4*u[3]+2*u[2]+u[1]
  Switch : Switch
  Switch1 : Switch
  Switch2 : Switch
  "N " : Outport
  wires:
  Switch2/1 -> Mux1/3
  Switch/1 -> Mux1/1
  Ualpha/1 -> Mux/1
  Ubeta/1 -> Mux/2
  Mux/1 -> B2/1, B1/1, B0/1
  B0/1 -> Switch/2
  B1/1 -> Switch1/2
  B2/1 -> Switch2/2
  Constant/1 -> Switch/1, Switch2/1, Switch1/1
  Constant1/1 -> Switch/3, Switch1/3, Switch2/3
  Switch1/1 -> Mux1/2
  Mux1/1 -> N/1
  N/1 -> "N "/1

== system MideaPMSM_V3_2019A/双闭环有感控制/MCU/SVPWMModel/时间切换点计算 ==
  N : Inport
  T1 : Inport  Port=2
  T2 : Inport  Port=3
  Tpwm : Inport  Port=4
  Fcn : Fcn  Expr=(u[3]-u[1]-u[2])/4
  Fcn1 : Fcn  Expr=(u[3]+u[1]-u[2])/4
  Fcn2 : Fcn  Expr=(u[3]+u[2]+u[1])/4
  Multiport Switch : MultiPortSwitch  Inputs=6
  Multiport Switch1 : MultiPortSwitch  Inputs=6
  Multiport Switch2 : MultiPortSwitch  Inputs=6
  Mux : Mux  Inputs=3
  Mux1 : Mux  Inputs=3
  Tcm1 Tcm2 Tcm3 : Outport
  wires:
  Mux/1 -> Fcn2/1, Fcn/1, Fcn1/1
  Tpwm/1 -> Mux/3
  T2/1 -> Mux/2
  T1/1 -> Mux/1
  Multiport Switch2/1 -> Mux1/3
  Multiport Switch1/1 -> Mux1/2
  Multiport Switch/1 -> Mux1/1
  Mux1/1 -> Tcm1 Tcm2 Tcm3/1
  Fcn/1 -> Multiport Switch/3, Multiport Switch/4, Multiport Switch1/6, Multiport Switch2/5, Multiport Switch2/7, Multiport Switch1/2
  Fcn1/1 -> Multiport Switch1/5, Multiport Switch2/3, Multiport Switch2/6, Multiport Switch1/4, Multiport Switch/7, Multiport Switch/2
  Fcn2/1 -> Multiport Switch/5, Multiport Switch/6, Multiport Switch1/3, Multiport Switch1/7, Multiport Switch2/2, Multiport Switch2/4
  N/1 -> Multiport Switch2/1, Multiport Switch1/1, Multiport Switch/1

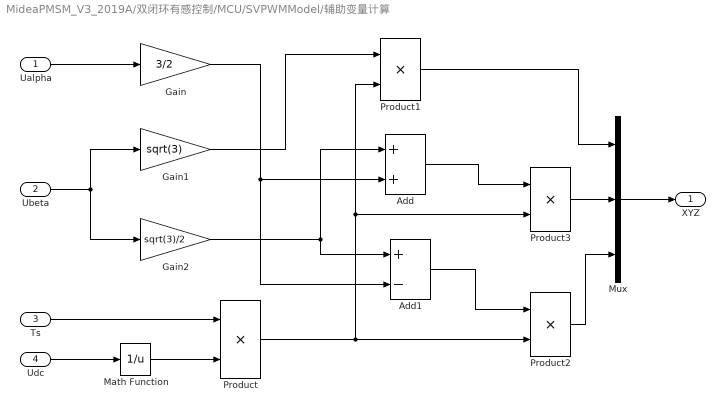
== system MideaPMSM_V3_2019A/双闭环有感控制/MCU/SVPWMModel/辅助变量计算 ==
  Ualpha : Inport
  Ubeta : Inport  Port=2
  Ts : Inport  Port=3
  Udc : Inport  Port=4
  Add : Sum
  Add1 : Sum  Inputs=+-
  Gain : Gain  Gain=3/2
  Gain1 : Gain  Gain=sqrt(3)
  Gain2 : Gain  Gain=sqrt(3)/2
  Math Function : Math  Operator=reciprocal  SaturateOnIntegerOverflow=on
  Mux : Mux  Inputs=3
  Product{,1..3} (4 alike) : Product  RndMeth=Zero
  XYZ : Outport
  wires:
  Mux/1 -> XYZ/1
  Product1/1 -> Mux/1
  Product3/1 -> Mux/2
  Product2/1 -> Mux/3
  Ualpha/1 -> Gain/1
  Ubeta/1 -> Gain2/1, Gain1/1
  Udc/1 -> Math Function/1
  Math Function/1 -> Product/2
  Ts/1 -> Product/1
  Gain1/1 -> Product1/1
  Product/1 -> Product2/2, Product1/2, Product3/2
  Gain/1 -> Add1/2, Add/2
  Gain2/1 -> Add/1, Add1/1
  Add1/1 -> Product2/1
  Add/1 -> Product3/1

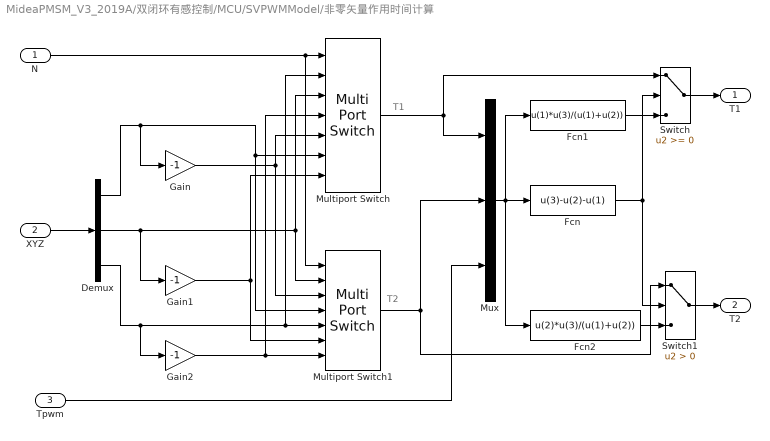
== system MideaPMSM_V3_2019A/双闭环有感控制/MCU/SVPWMModel/非零矢量作用时间计算 ==
  note: T1
  note: T2
  N : Inport
  XYZ : Inport  Port=2
  Tpwm : Inport  Port=3
  Demux : Demux  Outputs=3
  Fcn : Fcn  Expr=u(3)-u(2)-u(1)
  Fcn1 : Fcn  Expr=u(1)*u(3)/(u(1)+u(2))
  Fcn2 : Fcn  Expr=u(2)*u(3)/(u(1)+u(2))
  Gain : Gain  Gain=-1
  Gain1 : Gain  Gain=-1
  Gain2 : Gain  Gain=-1
  Multiport Switch : MultiPortSwitch  Inputs=6
  Multiport Switch1 : MultiPortSwitch  Inputs=6
  Mux : Mux  Inputs=3
  Switch : Switch
  Switch1 : Switch  Criteria=u2 > Threshold
  T1 : Outport
  T2 : Outport  Port=2
  wires:
  Tpwm/1 -> Mux/3
  XYZ/1 -> Demux/1
  Switch1/1 -> T2/1
  Switch/1 -> T1/1
  Fcn2/1 -> Switch1/3
  Fcn1/1 -> Switch/3
  Fcn/1 -> Switch/2, Switch1/2
  Mux/1 -> Fcn1/1, Fcn/1, Fcn2/1
  Multiport Switch/1 -> Switch/1, Mux/1
  Multiport Switch1/1 -> Switch1/1, Mux/2
  N/1 -> Multiport Switch/1, Multiport Switch1/1
  Demux/2 -> Multiport Switch/3, Multiport Switch1/2, Gain1/1
  Demux/3 -> Multiport Switch1/5, Multiport Switch/2, Gain2/1
  Demux/1 -> Multiport Switch/6, Multiport Switch1/4, Gain/1
  Gain/1 -> Multiport Switch1/3, Multiport Switch/5
  Gain2/1 -> Multiport Switch/4, Multiport Switch1/7
  Gain1/1 -> Multiport Switch1/6, Multiport Switch/7

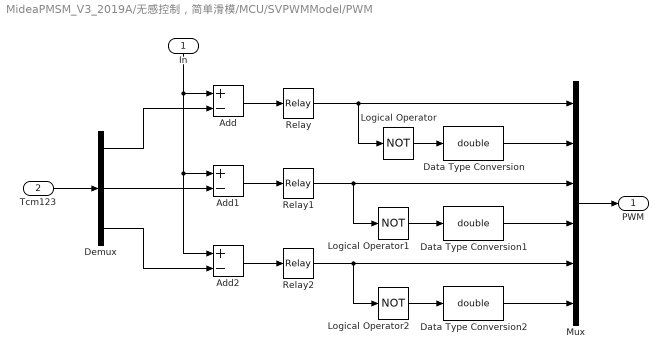
== system MideaPMSM_V3_2019A/无感控制，简单滑模/MCU/SVPWMModel/PWM ==
  In : Inport
  Tcm123 : Inport  Port=2
  Add : Sum  Inputs=+-
  Add1 : Sum  Inputs=+-
  Add2 : Sum  Inputs=+-
  Data Type Conversion : DataTypeConversion  OutDataTypeStr=double
  Data Type Conversion1 : DataTypeConversion  OutDataTypeStr=double
  Data Type Conversion2 : DataTypeConversion  OutDataTypeStr=double
  Demux : Demux  Outputs=3
  Logical Operator : Logic  Operator=NOT  AllPortsSameDT=off  OutDataTypeStr=boolean
  Logical Operator1 : Logic  Operator=NOT  AllPortsSameDT=off  OutDataTypeStr=boolean
  Logical Operator2 : Logic  Operator=NOT  AllPortsSameDT=off  OutDataTypeStr=boolean
  Mux : Mux  Inputs=6
  Relay : Relay  OffSwitchValue=-eps
  Relay1 : Relay  OffSwitchValue=-eps
  Relay2 : Relay  OffSwitchValue=-eps
  PWM : Outport
  wires:
  Demux/3 -> Add2/2
  Demux/2 -> Add1/2
  Demux/1 -> Add/2
  Relay2/1 -> Mux/5, Logical Operator2/1
  Relay1/1 -> Mux/3, Logical Operator1/1
  Relay/1 -> Logical Operator/1, Mux/1
  Mux/1 -> PWM/1
  Data Type Conversion/1 -> Mux/2
  Data Type Conversion1/1 -> Mux/4
  Data Type Conversion2/1 -> Mux/6
  Logical Operator2/1 -> Data Type Conversion2/1
  Logical Operator1/1 -> Data Type Conversion1/1
  Logical Operator/1 -> Data Type Conversion/1
  Add1/1 -> Relay1/1
  Add2/1 -> Relay2/1
  Add/1 -> Relay/1
  In/1 -> Add/1, Add2/1, Add1/1
  Tcm123/1 -> Demux/1

== system MideaPMSM_V3_2019A/无感控制，简单滑模/MCU/SVPWMModel/Sector Calculate ==
  Ualpha : Inport
  Ubeta : Inport  Port=2
  B0 : Fcn  Expr=u[2]
  B1 : Fcn  Expr=u[1]*sqrt(3/4)-0.5*u[2]
  B2 : Fcn  Expr=-u[1]*sqrt(3/4)-u[2]*0.5
  Constant : Constant
  Constant1 : Constant  Value=0
  Mux : Mux  Inputs=2
  Mux1 : Mux  Inputs=3
  N : Fcn  Expr=4*u[3]+2*u[2]+u[1]
  Switch : Switch
  Switch1 : Switch
  Switch2 : Switch
  "N " : Outport
  wires:
  Switch2/1 -> Mux1/3
  Switch/1 -> Mux1/1
  Ualpha/1 -> Mux/1
  Ubeta/1 -> Mux/2
  Mux/1 -> B2/1, B1/1, B0/1
  B0/1 -> Switch/2
  B1/1 -> Switch1/2
  B2/1 -> Switch2/2
  Constant/1 -> Switch/1, Switch2/1, Switch1/1
  Constant1/1 -> Switch/3, Switch1/3, Switch2/3
  Switch1/1 -> Mux1/2
  Mux1/1 -> N/1
  N/1 -> "N "/1

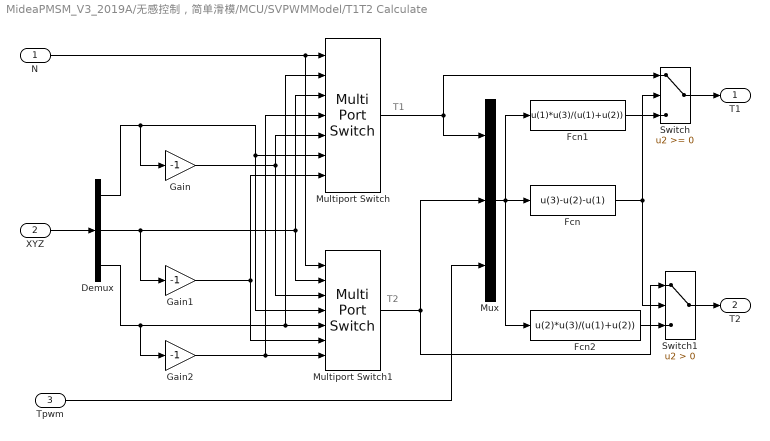
== system MideaPMSM_V3_2019A/无感控制，简单滑模/MCU/SVPWMModel/T1T2 Calculate ==
  note: T1
  note: T2
  N : Inport
  XYZ : Inport  Port=2
  Tpwm : Inport  Port=3
  Demux : Demux  Outputs=3
  Fcn : Fcn  Expr=u(3)-u(2)-u(1)
  Fcn1 : Fcn  Expr=u(1)*u(3)/(u(1)+u(2))
  Fcn2 : Fcn  Expr=u(2)*u(3)/(u(1)+u(2))
  Gain : Gain  Gain=-1
  Gain1 : Gain  Gain=-1
  Gain2 : Gain  Gain=-1
  Multiport Switch : MultiPortSwitch  Inputs=6
  Multiport Switch1 : MultiPortSwitch  Inputs=6
  Mux : Mux  Inputs=3
  Switch : Switch
  Switch1 : Switch  Criteria=u2 > Threshold
  T1 : Outport
  T2 : Outport  Port=2
  wires:
  Tpwm/1 -> Mux/3
  XYZ/1 -> Demux/1
  Switch1/1 -> T2/1
  Switch/1 -> T1/1
  Fcn2/1 -> Switch1/3
  Fcn1/1 -> Switch/3
  Fcn/1 -> Switch/2, Switch1/2
  Mux/1 -> Fcn1/1, Fcn/1, Fcn2/1
  Multiport Switch/1 -> Switch/1, Mux/1
  Multiport Switch1/1 -> Switch1/1, Mux/2
  N/1 -> Multiport Switch/1, Multiport Switch1/1
  Demux/2 -> Multiport Switch/3, Multiport Switch1/2, Gain1/1
  Demux/3 -> Multiport Switch1/5, Multiport Switch/2, Gain2/1
  Demux/1 -> Multiport Switch/6, Multiport Switch1/4, Gain/1
  Gain/1 -> Multiport Switch1/3, Multiport Switch/5
  Gain2/1 -> Multiport Switch/4, Multiport Switch1/7
  Gain1/1 -> Multiport Switch1/6, Multiport Switch/7

== system MideaPMSM_V3_2019A/无感控制，简单滑模/MCU/SVPWMModel/Tcm Calculate ==
  N : Inport
  T1 : Inport  Port=2
  T2 : Inport  Port=3
  Tpwm : Inport  Port=4
  Fcn : Fcn  Expr=(u[3]-u[1]-u[2])/4
  Fcn1 : Fcn  Expr=(u[3]+u[1]-u[2])/4
  Fcn2 : Fcn  Expr=(u[3]+u[2]+u[1])/4
  Multiport Switch : MultiPortSwitch  Inputs=6
  Multiport Switch1 : MultiPortSwitch  Inputs=6
  Multiport Switch2 : MultiPortSwitch  Inputs=6
  Mux : Mux  Inputs=3
  Mux1 : Mux  Inputs=3
  Tcm1 Tcm2 Tcm3 : Outport
  wires:
  Mux/1 -> Fcn2/1, Fcn/1, Fcn1/1
  Tpwm/1 -> Mux/3
  T2/1 -> Mux/2
  T1/1 -> Mux/1
  Multiport Switch2/1 -> Mux1/3
  Multiport Switch1/1 -> Mux1/2
  Multiport Switch/1 -> Mux1/1
  Mux1/1 -> Tcm1 Tcm2 Tcm3/1
  Fcn/1 -> Multiport Switch/3, Multiport Switch/4, Multiport Switch1/6, Multiport Switch2/5, Multiport Switch2/7, Multiport Switch1/2
  Fcn1/1 -> Multiport Switch1/5, Multiport Switch2/3, Multiport Switch2/6, Multiport Switch1/4, Multiport Switch/7, Multiport Switch/2
  Fcn2/1 -> Multiport Switch/5, Multiport Switch/6, Multiport Switch1/3, Multiport Switch1/7, Multiport Switch2/2, Multiport Switch2/4
  N/1 -> Multiport Switch2/1, Multiport Switch1/1, Multiport Switch/1

== system MideaPMSM_V3_2019A/无感控制，简单滑模/MCU/SVPWMModel/XYZ Calculate ==
  Ualpha : Inport
  Ubeta : Inport  Port=2
  Ts : Inport  Port=3
  Udc : Inport  Port=4
  Add : Sum
  Add1 : Sum  Inputs=+-
  Gain : Gain  Gain=3/2
  Gain1 : Gain  Gain=sqrt(3)
  Gain2 : Gain  Gain=sqrt(3)/2
  Math Function : Math  Operator=reciprocal  SaturateOnIntegerOverflow=on
  Mux : Mux  Inputs=3
  Product{,1..3} (4 alike) : Product  RndMeth=Zero
  XYZ : Outport
  wires:
  Mux/1 -> XYZ/1
  Product1/1 -> Mux/1
  Product3/1 -> Mux/2
  Product2/1 -> Mux/3
  Ualpha/1 -> Gain/1
  Ubeta/1 -> Gain2/1, Gain1/1
  Udc/1 -> Math Function/1
  Math Function/1 -> Product/2
  Ts/1 -> Product/1
  Gain1/1 -> Product1/1
  Product/1 -> Product2/2, Product1/2, Product3/2
  Gain/1 -> Add1/2, Add/2
  Gain2/1 -> Add/1, Add1/1
  Add1/1 -> Product2/1
  Add/1 -> Product3/1

== matlab function MideaPMSM_V3_2019A/无感控制，简单滑模/MCU/MATLAB Function ==
  data: Ualpha input; Pulse output; Ubeta input; Udc input; Tpwm input; trig input
function Pulse = SVPWM(Ualpha, Ubeta, Udc, Tpwm, trig)
N = SectorCaculate(Ualpha, Ubeta);
[T1, T2] = VectorTimeCaculate(Ualpha, Ubeta, Udc, Tpwm, N);
[Tcm1, Tcm2, Tcm3] = SwitchPoint(N, T1, T2, Tpwm);
[pwm1H, pwm1L, pwm2H, pwm2L, pwm3H, pwm3L] = PWMGen(Tcm1, Tcm2, Tcm3, trig);
Pulse = [pwm1H, pwm1L, pwm2H, pwm2L, pwm3H, pwm3L];

== matlab function MideaPMSM_V3_2019A/双闭环有感控制/MCU/MATLAB Function ==
  data: Ualpha input; Pulse output; Ubeta input; Udc input; Tpwm input; trig input
function Pulse = SVPWM(Ualpha, Ubeta, Udc, Tpwm, trig)
N = SectorCaculate(Ualpha, Ubeta);
[T1, T2] = VectorTimeCaculate(Ualpha, Ubeta, Udc, Tpwm, N);
[Tcm1, Tcm2, Tcm3] = SwitchPoint(N, T1, T2, Tpwm);
[pwm1H, pwm1L, pwm2H, pwm2L, pwm3H, pwm3L] = PWMGen(Tcm1, Tcm2, Tcm3, trig);
Pulse = [pwm1H, pwm1L, pwm2H, pwm2L, pwm3H, pwm3L];
